simulink model "TriggerLineFollow"  (R2023a)
settings: Solver=FixedStepDiscrete  StartTime=0.0  StopTime=15  FixedStep=0.01  RelTol=1e-3
undefined symbols (not defined in the file or in its folder): InputPWM, WheelSpeed
libraries: arduinolib x20, mobileRoboticsTrainingLib x2
settings Model: ExtModeTrigDuration=2  Creator=Boitumelo  LastModifiedBy=siyan
settings OptimizationCC: EnhancedBackFolding=on  PassReuseOutputArgsAs=Individual arguments  ZeroExternalMemoryAtStartup=off  ZeroInternalMemoryAtStartup=off  MaxStackSize=64  OptimizeBlockOrder=speed  DifferentSizesBufferReuse=on  OptimizationCustomize=off  EfficientTunableParamExpr=on
settings DebuggingCC: ParameterTunabilityLossMsg=error  UnconnectedInputMsg=warning  UnconnectedOutputMsg=warning  UnconnectedLineMsg=warning
settings HardwareCC: ProdBitPerPointer=32  ProdBitPerSizeT=32  ProdBitPerPtrDiffT=32  ProdLargestAtomicInteger=Long  ProdLargestAtomicFloat=Double  ProdWordSize=32  ProdHWDeviceType=ARM Compatible->ARM Cortex  UseEmbeddedCoderFeatures=off  UseSimulinkCoderFeatures=off
settings ModelReferenceCC: EnableRefExpFcnMdlSchedulingChecks=on
settings SFSimCC: MATLABDynamicMemAlloc=off
settings RTWCC: Description=Embedded Coder  SystemTargetFile=ert.tlc  HardwareBoard=Arduino Nano 33 IoT  TemplateMakefile=ert_default_tmf  Toolchain=Arduino ARM  BuildConfiguration=Faster Runs  DLArmComputeVersion=19.05
settings CodeAppCC: ForceParamTrailComments=on  IgnoreCustomStorageClasses=off  OperatorAnnotations=on  SimulinkDataObjDesc=on  SFDataObjDesc=on  InsertBlockDesc=on
settings ERTTargetCC: SupportContinuousTime=on  SupportNonInlinedSFcns=on  SupportVariableSizeSignals=on  ExtModeTransport=3  ExtModeStaticAlloc=on  ExtModeAutomaticAllocSize=off  ExtModeStaticAllocSize=8192  ExtModeMexFile=ext_xcp  ExtModeIntrfLevel=Level2 - Open

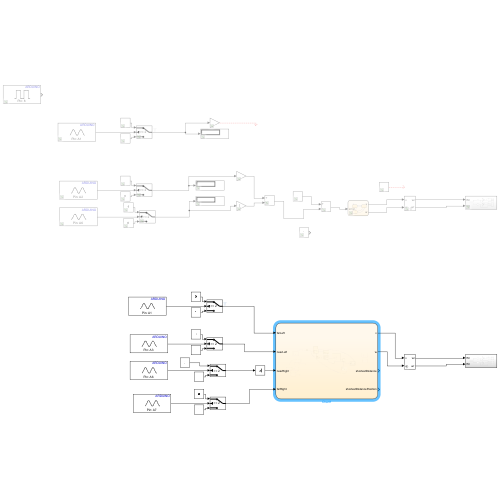
[thumbnail: Simulink's stored preview of the top-level diagram]
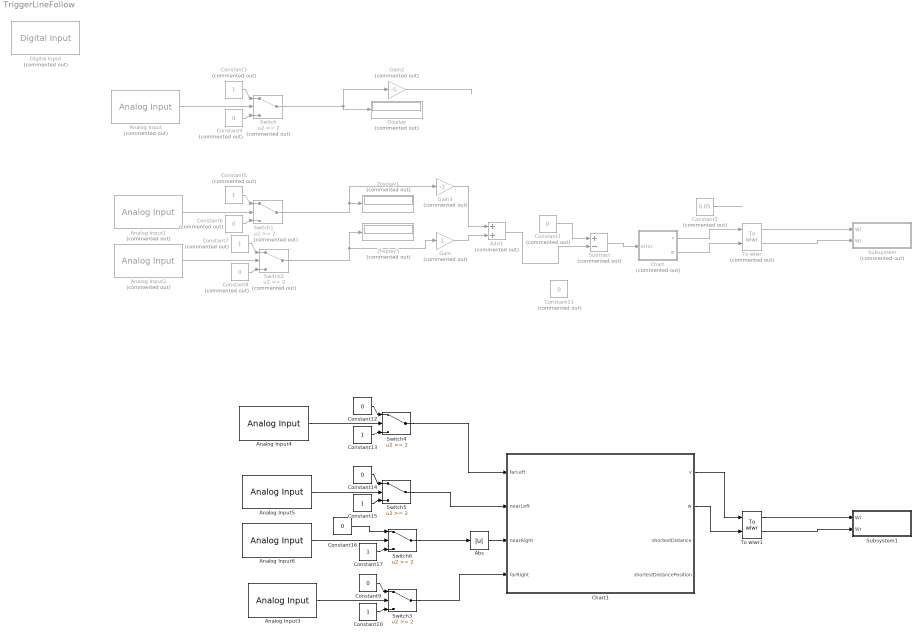
== system TriggerLineFollow ==
  Abs : Abs  SaturateOnIntegerOverflow=off
  Add1 : Sum  Commented=on
  Analog Input : arduinolib/Analog Input  Commented=on  pinNumber=1  ReadResultsOnly=off  ConversionTriggerSource=Software  ExternalTriggerType=uint32( 0 )  OutputDataType=uint16  EnableConversionCompleteNotify=off  EnableOuputStatus=off  SampleTime=-1  blockPlatform=arduino
  Analog Input1 : arduinolib/Analog Input  Commented=on  pinNumber=2  ReadResultsOnly=off  ConversionTriggerSource=Software  ExternalTriggerType=uint32( 0 )  OutputDataType=uint16  EnableConversionCompleteNotify=off  EnableOuputStatus=off  SampleTime=-1  blockPlatform=arduino
  Analog Input2 : arduinolib/Analog Input  Commented=on  pinNumber=6  ReadResultsOnly=off  ConversionTriggerSource=Software  ExternalTriggerType=uint32( 0 )  OutputDataType=uint16  EnableConversionCompleteNotify=off  EnableOuputStatus=off  SampleTime=-1  blockPlatform=arduino
  Analog Input3 : arduinolib/Analog Input  pinNumber=7  ReadResultsOnly=off  ConversionTriggerSource=Software  ExternalTriggerType=uint32( 0 )  OutputDataType=uint16  EnableConversionCompleteNotify=off  EnableOuputStatus=off  SampleTime=-1  blockPlatform=arduino
  Analog Input4 : arduinolib/Analog Input  pinNumber=1  ReadResultsOnly=off  ConversionTriggerSource=Software  ExternalTriggerType=uint32( 0 )  OutputDataType=uint16  EnableConversionCompleteNotify=off  EnableOuputStatus=off  SampleTime=-1  blockPlatform=arduino
  Analog Input5 : arduinolib/Analog Input  pinNumber=3  ReadResultsOnly=off  ConversionTriggerSource=Software  ExternalTriggerType=uint32( 0 )  OutputDataType=uint16  EnableConversionCompleteNotify=off  EnableOuputStatus=off  SampleTime=-1  blockPlatform=arduino
  Analog Input6 : arduinolib/Analog Input  pinNumber=6  ReadResultsOnly=off  ConversionTriggerSource=Software  ExternalTriggerType=uint32( 0 )  OutputDataType=uint16  EnableConversionCompleteNotify=off  EnableOuputStatus=off  SampleTime=-1  blockPlatform=arduino
  Chart : Stateflow chart  Commented=on  TreatAsAtomicUnit=on
  Chart1 : Stateflow chart  TreatAsAtomicUnit=on
  Constant{1,4,6,8,11} (5 alike) : Constant  Commented=on  Value=0
  Constant{10,13,15,17} (4 alike) : Constant
  Constant{9,12,14,16} (4 alike) : Constant  Value=0
  Constant2 : Constant  Commented=on  Value=0.05
  Constant3 : Constant  Commented=on
  Constant5 : Constant  Commented=on
  Constant7 : Constant  Commented=on
  Digital Input : arduinolib/Digital Input  Commented=on  pinNumber=8  mode=Default  Direction=input  SampleTime=0.1  blockPlatform=arduino
  Display : Display  Commented=on
  Display1 : Display  Commented=on
  Display3 : Display  Commented=on
  Gain : Gain  Commented=on
  Gain2 : Gain  Commented=on  Gain=-5
  Gain3 : Gain  Commented=on  Gain=-1
  Subsystem : Subsystem  Commented=on
      settings: LibrarySourceBlock=|
      | hdlsllib/Ports &
      | Subsystems/Subsystem
  Subsystem1 : Subsystem
      settings: LibrarySourceBlock=|
      | hdlsllib/Ports &
      | Subsystems/Subsystem
  Subtract : Sum  Commented=on  Inputs=+-
  Switch : Switch  Commented=on  Threshold=2  SaturateOnIntegerOverflow=off  InputSameDT=off
  Switch1 : Switch  Commented=on  Threshold=2  SaturateOnIntegerOverflow=off  InputSameDT=off
  Switch2 : Switch  Commented=on  Threshold=2  SaturateOnIntegerOverflow=off  InputSameDT=off
  Switch{3..6} (4 alike) : Switch  Threshold=2  SaturateOnIntegerOverflow=off  InputSameDT=off
  To wlwr : mobileRoboticsTrainingLib/To wlwr  Commented=on  axleLength=axleLength  wheelR=wheelR
      link override change parameters: Gain=[1 +axleLength/2; 1 -axleLength/2]
  To wlwr1 : mobileRoboticsTrainingLib/To wlwr  axleLength=axleLength  wheelR=wheelR
      link override change parameters: Gain=[1 +axleLength/2; 1 -axleLength/2]
  wires:
  Switch/1 -> Gain2/1, Display/1
  Switch1/1 -> Gain3/1, Display1/1
  Switch2/1 -> Display3/1, Gain/1
  Gain2/1 -> ?
  Constant1/1 -> Subtract/1
  Add1/1 -> Subtract/2
  Constant2/1 -> ?
  Subtract/1 -> Chart/1(error)
  Chart/2(w) -> To wlwr/2
  Gain3/1 -> Add1/1
  To wlwr/1 -> Subsystem/1(Wl)
  To wlwr/2 -> Subsystem/2(Wr)
  Analog Input/1 -> Switch/2
  Constant3/1 -> Switch/1
  Constant4/1 -> Switch/3
  Constant5/1 -> Switch1/1
  Constant6/1 -> Switch1/3
  Analog Input1/1 -> Switch1/2
  Constant7/1 -> Switch2/1
  Constant8/1 -> Switch2/3
  Analog Input2/1 -> Switch2/2
  Constant9/1 -> Switch3/1
  Constant10/1 -> Switch3/3
  Analog Input3/1 -> Switch3/2
  Gain/1 -> Add1/2
  Chart/1(v) -> To wlwr/1
  Analog Input6/1 -> Switch6/2
  Constant17/1 -> Switch6/3
  Constant15/1 -> Switch5/3
  Constant16/1 -> Switch6/1
  Constant13/1 -> Switch4/3
  Analog Input5/1 -> Switch5/2
  Constant14/1 -> Switch5/1
  Constant12/1 -> Switch4/1
  Analog Input4/1 -> Switch4/2
  Switch4/1 -> Chart1/1(farLeft)
  Switch5/1 -> Chart1/2(nearLeft)
  Switch3/1 -> Chart1/4(farRight)
  To wlwr1/1 -> Subsystem1/1(Wl)
  To wlwr1/2 -> Subsystem1/2(Wr)
  Chart1/1(v) -> To wlwr1/1
  Chart1/2(w) -> To wlwr1/2
  Switch6/1 -> Abs/1
  Abs/1 -> Chart1/3(nearRight)

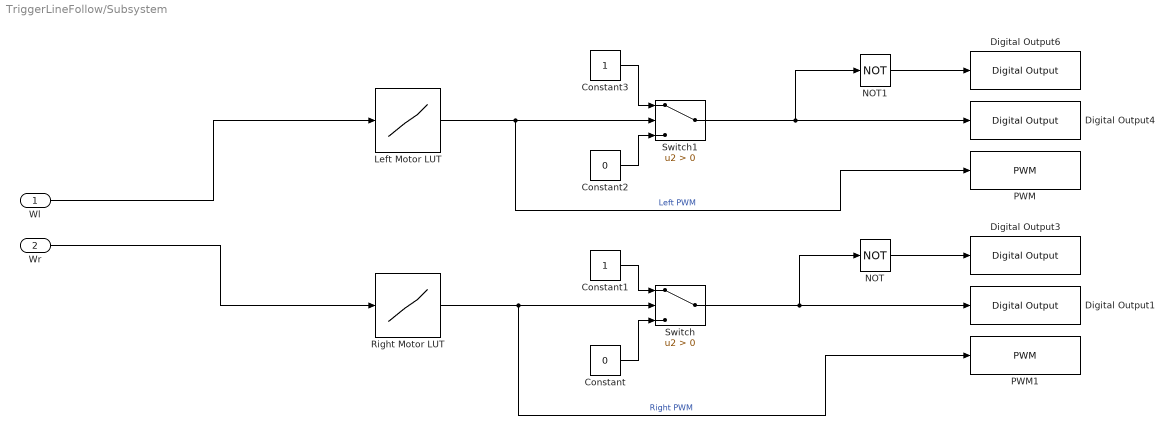
== system TriggerLineFollow/Subsystem ==
  Wl : Inport
  Wr : Inport  Port=2
  Constant : Constant  Value=0
  Constant1 : Constant
  Constant2 : Constant  Value=0
  Constant3 : Constant
  Digital Output1 : arduinolib/Digital Output  pinNumber=8  Direction=output  blockPlatform=arduino
  Digital Output3 : arduinolib/Digital Output  pinNumber=11  Direction=output  blockPlatform=arduino
  Digital Output4 : arduinolib/Digital Output  pinNumber=13  Direction=output  blockPlatform=arduino
  Digital Output6 : arduinolib/Digital Output  pinNumber=12  Direction=output  blockPlatform=arduino
  Left Motor LUT : Lookup_n-D  NumberOfTableDimensions=1  BreakpointsForDimension1=WheelSpeed  Table=InputPWM  InterpMethod=Nearest  ExtrapMethod=Clip  InternalRulePriority=Speed  RndMeth=Simplest
  NOT : Logic  Operator=NOT  IconShape=distinctive  AllPortsSameDT=off  OutDataTypeStr=boolean
  NOT1 : Logic  Operator=NOT  IconShape=distinctive  AllPortsSameDT=off  OutDataTypeStr=boolean
  PWM : arduinolib/PWM  pinNumber=9  frequencyType=Default  desiredFrequency=490.2  achievableFrequency=490.2
  PWM1 : arduinolib/PWM  pinNumber=10  frequencyType=Default  desiredFrequency=490.2  achievableFrequency=490.2
  Right Motor LUT : Lookup_n-D  NumberOfTableDimensions=1  BreakpointsForDimension1=WheelSpeed  Table=InputPWM  InterpMethod=Nearest  ExtrapMethod=Clip  InternalRulePriority=Speed  RndMeth=Simplest
  Switch : Switch  Criteria=u2 > Threshold  SaturateOnIntegerOverflow=off  InputSameDT=off
  Switch1 : Switch  Criteria=u2 > Threshold  SaturateOnIntegerOverflow=off  InputSameDT=off
  wires:
  Wr/1 -> Right Motor LUT/1
  Wl/1 -> Left Motor LUT/1
  Right Motor LUT/1 -> PWM1/1, Switch/2  "Right PWM"
  Left Motor LUT/1 -> PWM/1, Switch1/2  "Left PWM"
  NOT1/1 -> Digital Output6/1
  Constant1/1 -> Switch/1
  Constant/1 -> Switch/3
  Constant2/1 -> Switch1/3
  Constant3/1 -> Switch1/1
  Switch/1 -> NOT/1, Digital Output1/1
  Switch1/1 -> NOT1/1, Digital Output4/1
  NOT/1 -> Digital Output3/1

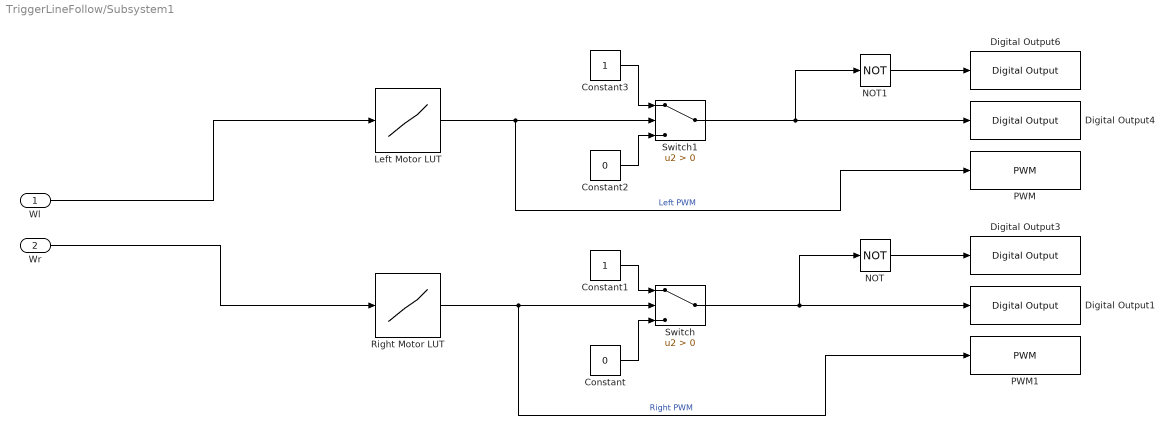
== system TriggerLineFollow/Subsystem1 ==
  Wl : Inport
  Wr : Inport  Port=2
  Constant : Constant  Value=0
  Constant1 : Constant
  Constant2 : Constant  Value=0
  Constant3 : Constant
  Digital Output1 : arduinolib/Digital Output  pinNumber=8  Direction=output  blockPlatform=arduino
  Digital Output3 : arduinolib/Digital Output  pinNumber=11  Direction=output  blockPlatform=arduino
  Digital Output4 : arduinolib/Digital Output  pinNumber=13  Direction=output  blockPlatform=arduino
  Digital Output6 : arduinolib/Digital Output  pinNumber=12  Direction=output  blockPlatform=arduino
  Left Motor LUT : Lookup_n-D  NumberOfTableDimensions=1  BreakpointsForDimension1=WheelSpeed  Table=InputPWM  InterpMethod=Nearest  ExtrapMethod=Clip  InternalRulePriority=Speed  RndMeth=Simplest
  NOT : Logic  Operator=NOT  IconShape=distinctive  AllPortsSameDT=off  OutDataTypeStr=boolean
  NOT1 : Logic  Operator=NOT  IconShape=distinctive  AllPortsSameDT=off  OutDataTypeStr=boolean
  PWM : arduinolib/PWM  pinNumber=9  frequencyType=Default  desiredFrequency=490.2  achievableFrequency=490.2
  PWM1 : arduinolib/PWM  pinNumber=10  frequencyType=Default  desiredFrequency=490.2  achievableFrequency=490.2
  Right Motor LUT : Lookup_n-D  NumberOfTableDimensions=1  BreakpointsForDimension1=WheelSpeed  Table=InputPWM  InterpMethod=Nearest  ExtrapMethod=Clip  InternalRulePriority=Speed  RndMeth=Simplest
  Switch : Switch  Criteria=u2 > Threshold  SaturateOnIntegerOverflow=off  InputSameDT=off
  Switch1 : Switch  Criteria=u2 > Threshold  SaturateOnIntegerOverflow=off  InputSameDT=off
  wires:
  Wr/1 -> Right Motor LUT/1
  Wl/1 -> Left Motor LUT/1
  Right Motor LUT/1 -> PWM1/1, Switch/2  "Right PWM"
  Left Motor LUT/1 -> PWM/1, Switch1/2  "Left PWM"
  NOT1/1 -> Digital Output6/1
  Constant1/1 -> Switch/1
  Constant/1 -> Switch/3
  Constant2/1 -> Switch1/3
  Constant3/1 -> Switch1/1
  Switch/1 -> NOT/1, Digital Output1/1
  Switch1/1 -> NOT1/1, Digital Output4/1
  NOT/1 -> Digital Output3/1

== stateflow chart TriggerLineFollow/Chart1 ==
  state Initialisation
    entry:
    numBranches = 0
    shortestDistance = 10 %No Object will be 10m away just used as reference
    shortestDistancePosition =0
  state LineFollowingOnMainLine
    entry:
    v = 0.1
    w= 0
    state Neutral
      entry: w = 0
    state TurnLeft
      entry:
      w = 1
    state TurnRight
      entry:
      w = -1
    (default) -> LineFollowingOnMainLine.Neutral
    LineFollowingOnMainLine.Neutral -> LineFollowingOnMainLine.TurnLeft [order 2] : [nearRight ==0]
    LineFollowingOnMainLine.TurnLeft -> LineFollowingOnMainLine.Neutral : [nearRight ==1]
    LineFollowingOnMainLine.TurnRight -> LineFollowingOnMainLine.Neutral : [nearLeft ==1]
    LineFollowingOnMainLine.Neutral -> LineFollowingOnMainLine.TurnRight [order 1] : [nearLeft ==0]
  state EndOfMaze
    entry:
    v=0
    w=0
  state RotateRightBranch
    entry:
    v=0
    w=-1.5
    leftBranch = false
    state Rotate
      entry:
      w= -1.5
    state ContinueRotateAndSeekNewLine
      entry:
      w= -1.5
    state StopAndReturn
      entry:
      w = 0
    (default) -> RotateRightBranch.Rotate
    (default) -> RotateRightBranch.Rotate [commented out]
    RotateRightBranch.Rotate -> RotateRightBranch.ContinueRotateAndSeekNewLine : [after(2,sec)&&(nearLeft ==0 || nearRight ==0)]
    RotateRightBranch.ContinueRotateAndSeekNewLine -> RotateRightBranch.StopAndReturn : [nearLeft ==1 && nearRight ==1]
  state TurnBackToMazeToFindShortestObject1 [commented out]
    entry:
    v=0
    w=-1.5
    numLinesToPass = numBranches-shortestDistancePosition
    state Rotate [commented out]
      entry:
      w= -1.5
    state ContinueRotateAndSeekNewLine [commented out]
      entry:
      w= -1.5
    state StopAndReturn [commented out]
      entry:
      w = 0
    (default) -> TurnBackToMazeToFindShortestObject1.Rotate [commented out]
    (default) -> TurnBackToMazeToFindShortestObject1.Rotate [commented out]
    TurnBackToMazeToFindShortestObject1.Rotate -> TurnBackToMazeToFindShortestObject1.ContinueRotateAndSeekNewLine [commented out] : [after(2,sec)&&(nearLeft ==0 || nearRight ==0)]
    TurnBackToMazeToFindShortestObject1.ContinueRotateAndSeekNewLine -> TurnBackToMazeToFindShortestObject1.StopAndReturn [commented out] : [nearLeft ==1 && nearRight ==1]
  state StopAndDetect
    entry:
    v=0
    w=0
    numBranches = numBranches + 1
    state MeasureAndStoreDistance [commented out]
      %Measure the distance using ultrasonic sensor
      %using variable currentDistance and light up LED
    state UpdateClosestDistance [commented out]
      %Onlyupdates if shorter distance else carries on
      entry:
      shortestDistancePosition = numObjects
      shortestDistance = distance
    (default) -> MeasureAndStoreDistance [commented out]
    MeasureAndStoreDistance -> UpdateClosestDistance [commented out] : [distance < shortestDistance]
  state TurnBackToMaze [commented out]
    entry:
    v=0
    w=-1.5
    state Rotate [commented out]
      entry:
      w= -1.5
    state ContinueRotateAndSeekNewLine [commented out]
      entry:
      w= -1.5
    state StopAndReturn [commented out]
      entry:
      w = 0
    (default) -> TurnBackToMaze.Rotate [commented out]
    (default) -> TurnBackToMaze.Rotate [commented out]
    TurnBackToMaze.Rotate -> TurnBackToMaze.ContinueRotateAndSeekNewLine [commented out] : [after(2,sec)&&(nearLeft ==0 || nearRight ==0)]
    TurnBackToMaze.ContinueRotateAndSeekNewLine -> TurnBackToMaze.StopAndReturn [commented out] : [nearLeft ==1 && nearRight ==1]
  state RotateLeftBranch
    entry:
    v=0
    w=1.5
    leftBranch = true
    state Rotate
      entry:
      w= 1.5
    state ContinueRotateAndSeekNewLine
      entry:
      w= 1.5
    state StopAndReturn
      entry:
      w = 0
    (default) -> RotateLeftBranch.Rotate
    RotateLeftBranch.Rotate -> RotateLeftBranch.ContinueRotateAndSeekNewLine : [after(2,sec)&&(nearLeft ==0 || nearRight ==0)]
    RotateLeftBranch.ContinueRotateAndSeekNewLine -> RotateLeftBranch.StopAndReturn : [nearLeft ==1 && nearRight ==1]
  state OnBranchLineFollowing
    entry:
    v = 0.1
    w= 0
    state Neutral
      entry: w = 0
    state TurnLeft
      entry:
      w = 1
    state TurnRight
      entry:
      w = -1
    (default) -> OnBranchLineFollowing.Neutral
    OnBranchLineFollowing.Neutral -> OnBranchLineFollowing.TurnLeft [order 2] : [nearRight ==0]
    OnBranchLineFollowing.TurnLeft -> OnBranchLineFollowing.Neutral : [nearRight ==1]
    OnBranchLineFollowing.TurnRight -> OnBranchLineFollowing.Neutral : [nearLeft ==1]
    OnBranchLineFollowing.Neutral -> OnBranchLineFollowing.TurnRight [order 1] : [nearLeft ==0]
  state LineFollowingOnMainLineToFindShortest [commented out]
    entry:
    v = 0.1
    w= 0
    state Neutral [commented out]
      entry: w = 0
    state TurnLeft [commented out]
      entry:
      w = 1
    state TurnRight [commented out]
      entry:
      w = -1
    (default) -> LineFollowingOnMainLineToFindShortest.Neutral [commented out]
    LineFollowingOnMainLineToFindShortest.Neutral -> LineFollowingOnMainLineToFindShortest.TurnLeft [commented out] : [nearRight ==0]
    LineFollowingOnMainLineToFindShortest.TurnLeft -> LineFollowingOnMainLineToFindShortest.Neutral [commented out] : [nearRight ==1]
    LineFollowingOnMainLineToFindShortest.TurnRight -> LineFollowingOnMainLineToFindShortest.Neutral [commented out] : [nearLeft ==1]
    LineFollowingOnMainLineToFindShortest.Neutral -> LineFollowingOnMainLineToFindShortest.TurnRight [commented out] : [nearLeft ==0]
  state ReturnToMainLineBranchLineFollowing [commented out]
    entry:
    v = 0.1
    w= 0
    state Neutral [commented out]
      entry: w = 0
    state TurnLeft [commented out]
      entry:
      w = 1
    state TurnRight [commented out]
      entry:
      w = -1
    (default) -> ReturnToMainLineBranchLineFollowing.Neutral [commented out]
    ReturnToMainLineBranchLineFollowing.Neutral -> ReturnToMainLineBranchLineFollowing.TurnLeft [commented out] : [nearRight ==0]
    ReturnToMainLineBranchLineFollowing.TurnLeft -> ReturnToMainLineBranchLineFollowing.Neutral [commented out] : [nearRight ==1]
    ReturnToMainLineBranchLineFollowing.TurnRight -> ReturnToMainLineBranchLineFollowing.Neutral [commented out] : [nearLeft ==1]
    ReturnToMainLineBranchLineFollowing.Neutral -> ReturnToMainLineBranchLineFollowing.TurnRight [commented out] : [nearLeft ==0]
  state MoveBackwardsTowardsMainLine
    entry:
    v=-0.1
    w=0
  state RotateLeftBackToMain
    entry:
    v=0
    w=1.5
    state Rotate
      entry:
      w= -1.5
    state ContinueRotateAndSeekNewLine
      entry:
      w= -1.5
    state StopAndReturn
      entry:
      w = 0
    (default) -> RotateLeftBackToMain.Rotate
    (default) -> RotateLeftBackToMain.Rotate [commented out]
    RotateLeftBackToMain.Rotate -> RotateLeftBackToMain.ContinueRotateAndSeekNewLine : [after(2,sec)&&(nearLeft ==0 || nearRight ==0)]
    RotateLeftBackToMain.ContinueRotateAndSeekNewLine -> RotateLeftBackToMain.StopAndReturn : [nearLeft ==1 && nearRight ==1]
  state DeadEnd
    entry:
    v = 0
    w=0
    numBranches = numBranches +1
  state DecrementNumLinesToPass [commented out]
    numLinesToPass = numLinesToPass -1
    %Note I included the after 3 sec in the
    %condition as debouncing to prevent the same branch being measured twice
    %Going to assume two branches are not close enough to be travelled in three seconds
  state RotateRightBackToMain
    entry:
    v=0
    w=-1.5
    state Rotate
      entry:
      w= 1.5
    state ContinueRotateAndSeekNewLine
      entry:
      w= 1.5
    state StopAndReturn
      entry:
      w = 0
    (default) -> RotateRightBackToMain.Rotate
    (default) -> RotateRightBackToMain.Rotate [commented out]
    RotateRightBackToMain.Rotate -> RotateRightBackToMain.ContinueRotateAndSeekNewLine : [after(2,sec)&&(nearLeft ==0 || nearRight ==0)]
    RotateRightBackToMain.ContinueRotateAndSeekNewLine -> RotateRightBackToMain.StopAndReturn : [nearLeft ==1 && nearRight ==1]
  state RotateLeftBranchToClosestObject [commented out]
    entry:
    v=0
    w=1.5
    state Rotate [commented out]
      entry:
      w= 1.5
    state ContinueRotateAndSeekNewLine [commented out]
      entry:
      w= 1.5
    state StopAndReturn [commented out]
      entry:
      w = 0
    (default) -> RotateLeftBranchToClosestObject.Rotate [commented out]
    RotateLeftBranchToClosestObject.Rotate -> RotateLeftBranchToClosestObject.ContinueRotateAndSeekNewLine [commented out] : [after(2,sec)&&(nearLeft ==0 || nearRight ==0)]
    RotateLeftBranchToClosestObject.ContinueRotateAndSeekNewLine -> RotateLeftBranchToClosestObject.StopAndReturn [commented out] : [nearLeft ==1 && nearRight ==1]
  state RotateRightBranchToClosestObject [commented out]
    entry:
    v=0
    w=-1.5
    leftBranch = false
    state Rotate [commented out]
      entry:
      w= -1.5
    state ContinueRotateAndSeekNewLine [commented out]
      entry:
      w= -1.5
    state StopAndReturn [commented out]
      entry:
      w = 0
    (default) -> RotateRightBranchToClosestObject.Rotate [commented out]
    (default) -> RotateRightBranchToClosestObject.Rotate [commented out]
    RotateRightBranchToClosestObject.Rotate -> RotateRightBranchToClosestObject.ContinueRotateAndSeekNewLine [commented out] : [after(2,sec)&&(nearLeft ==0 || nearRight ==0)]
    RotateRightBranchToClosestObject.ContinueRotateAndSeekNewLine -> RotateRightBranchToClosestObject.StopAndReturn [commented out] : [nearLeft ==1 && nearRight ==1]
  state ShortestObjectBranchLineFollowing [commented out]
    entry:
    v = 0.1
    w= 0
    state Neutral [commented out]
      entry: w = 0
    state TurnLeft [commented out]
      entry:
      w = 1
    state TurnRight [commented out]
      entry:
      w = -1
    (default) -> ShortestObjectBranchLineFollowing.Neutral [commented out]
    ShortestObjectBranchLineFollowing.Neutral -> ShortestObjectBranchLineFollowing.TurnLeft [commented out] : [nearRight ==0]
    ShortestObjectBranchLineFollowing.TurnLeft -> ShortestObjectBranchLineFollowing.Neutral [commented out] : [nearRight ==1]
    ShortestObjectBranchLineFollowing.TurnRight -> ShortestObjectBranchLineFollowing.Neutral [commented out] : [nearLeft ==1]
    ShortestObjectBranchLineFollowing.Neutral -> ShortestObjectBranchLineFollowing.TurnRight [commented out] : [nearLeft ==0]
  state StopAtClosestObject [commented out]
    entry:
    v=0
    w=0
  (default) -> Initialisation
  Initialisation -> LineFollowingOnMainLine
  RotateLeftBackToMain.StopAndReturn -> LineFollowingOnMainLine : [after(1,sec)]
  EndOfMaze -> TurnBackToMazeToFindShortestObject1 [commented out] : [after(7,sec)]
  LineFollowingOnMainLine -> EndOfMaze [order 3] : [farLeft==1 && nearLeft ==1 && nearRight==1 && farRight ==1]
  LineFollowingOnMainLine -> RotateRightBranch [order 2] : [farLeft==0 && nearLeft ==1 && nearRight==1 && farRight ==1]
  RotateRightBackToMain.StopAndReturn -> LineFollowingOnMainLine : [after(1,sec)]
  LineFollowingOnMainLine -> RotateLeftBranch [order 1] : [farLeft==1 && nearLeft ==1 && nearRight==1 && farRight ==0]
  RotateRightBranch.StopAndReturn -> OnBranchLineFollowing : [after(1,sec)]
  TurnBackToMazeToFindShortestObject1.StopAndReturn -> LineFollowingOnMainLineToFindShortest [commented out] : [after(1,sec)]
  TurnBackToMaze.StopAndReturn -> ReturnToMainLineBranchLineFollowing [commented out] : [after(1,sec)]
  RotateLeftBranch.StopAndReturn -> OnBranchLineFollowing : [after(1,sec)]
  OnBranchLineFollowing -> StopAndDetect [order 1] : [farLeft==1 && farRight ==1]
  StopAndDetect -> MoveBackwardsTowardsMainLine : [after(3,sec)]
  LineFollowingOnMainLineToFindShortest -> RotateLeftBranchToClosestObject [commented out] : [numLinesToPass==0 &&after(2,sec)&& (farLeft==1 && nearLeft ==1 && nearRight==1 && farRight ==0)]
  LineFollowingOnMainLineToFindShortest -> DecrementNumLinesToPass [commented out] : [numLinesToPass>0 &&after(2,sec)&& ((farLeft==1 && nearLeft ==1 && nearRight==1 && farRight ==0) || (farLeft==0 && nearLeft ==1 && nearRight==1 && farRight ==1))]
  OnBranchLineFollowing -> DeadEnd [order 2] : [farLeft ==0 && nearLeft==0 && nearRight ==0&&farRight == 0]
  DeadEnd -> MoveBackwardsTowardsMainLine : [after(1,sec)]
  MoveBackwardsTowardsMainLine -> RotateRightBackToMain [order 2] : [leftBranch && farLeft==1 && farRight ==1]
  MoveBackwardsTowardsMainLine -> RotateLeftBackToMain [order 1] : [~leftBranch && farLeft==1 && farRight ==1]
  LineFollowingOnMainLineToFindShortest -> RotateRightBranchToClosestObject [commented out] : [numLinesToPass==0 &&after(2,sec)&& (farLeft==0 && nearLeft ==1 && nearRight==1 && farRight ==1)]
  DecrementNumLinesToPass -> LineFollowingOnMainLineToFindShortest [commented out]
  RotateLeftBranchToClosestObject.StopAndReturn -> ShortestObjectBranchLineFollowing [commented out] : [after(1,sec)]
  RotateRightBranchToClosestObject.StopAndReturn -> ShortestObjectBranchLineFollowing [commented out] : [after(1,sec)]
  ShortestObjectBranchLineFollowing -> StopAtClosestObject [commented out] : [farLeft==1 && farRight ==1]
  data: farLeft input; nearLeft input; nearRight input; farRight input; v output; w output; shortestDistance output; shortestDistancePosition output; numBranches local; leftBranch local

== stateflow chart TriggerLineFollow/Chart ==
  state Straight
    entry:
    w =0
    v= 0.06
  state SteerRight
    entry:
    w = -1
    v=0.045
  state SteerLeft
    entry:
    w= 3.8
    v=0.045
  (default) -> Straight
  Straight -> SteerRight [order 1] : [error > 0.1]
  SteerRight -> Straight [order 1] : [error <0.1]
  Straight -> SteerLeft [order 2] : [error <-0.1]
  SteerLeft -> Straight [order 1] : [error >  -0.1]
  SteerLeft -> SteerRight [order 2] : [error>0.1]
  SteerRight -> SteerLeft [order 2] : [error < -0.1]
  data: v output; error input; w output
